simulink model "mariner_simtr"  (R2018b)
settings: Solver=FixedStepAuto  StartTime=0.0  StopTime=600  FixedStep=0.1  RelTol=1e-3
libraries: neural x211, simulink x2
(part 10 of 10)

== system mariner_simtr/NN transform (normalizing)/Layer 4/Delays 1 ==
  "p{4}" : Inport  PortDimensions=24
      mask Display: e = 0.06;c1 = [120 230 180]/255;c2 = ([120 230 180]+0)/(256+128);c3 = ([120 230 180]+128)/(256+128);patch([0 1 1 0],[0 0 1 1],c1);patch([0 1 1 1-e 1-e 0+e],[0 0 1 1-e 0+e 0+e],c2);patch([0 0 1 1-e 0+e 0+e],[0 1 1 1-e 1-e 0+e],c3);plot([0 1 1 0 0],[0 0 1 1 0]);
  mux : Mux  Inputs=1
      mask Display: e = 0.06;c1 = [120 150 230]/255;c2 = ([120 150 230]+0)/383;c3 = ([120 150 230]+128)/383;patch([0 1 1 0],[0 0 1 1],c1);patch([0 1 1 1-e 1-e 0+e],[0 0 1 1-e 0+e 0+e],c2);patch([0 0 1 1-e 0+e 0+e],[0 1 1 1-e 1-e 0+e],c3);plot([0 1 1 0 0],[0 0 1 1 0]);disp('Mux')
  "pd{4,3}" : Outport
      mask Display: e = 0.06;c1 = [120 230 180]/255;c2 = ([120 230 180]+0)/(256+128);c3 = ([120 230 180]+128)/(256+128);patch([0 1 1 0],[0 0 1 1],c1);patch([0 1 1 1-e 1-e 0+e],[0 0 1 1-e 0+e 0+e],c2);patch([0 0 1 1-e 0+e 0+e],[0 1 1 1-e 1-e 0+e],c3);plot([0 1 1 0 0],[0 0 1 1 0]);
  wires:
  mux/1 -> "pd{4,3}"/1
  "p{4}"/1 -> mux/1

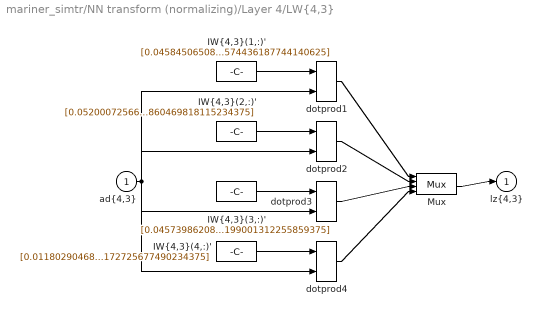
== system mariner_simtr/NN transform (normalizing)/Layer 4/LW{4,3} ==
  "ad{4,3}" : Inport  PortDimensions=24
      mask Display: e = 0.06;c1 = [120 230 180]/255;c2 = ([120 230 180]+0)/(256+128);c3 = ([120 230 180]+128)/(256+128);patch([0 1 1 0],[0 0 1 1],c1);patch([0 1 1 1-e 1-e 0+e],[0 0 1 1-e 0+e 0+e],c2);patch([0 0 1 1-e 0+e 0+e],[0 1 1 1-e 1-e 0+e],c3);plot([0 1 1 0 0],[0 0 1 1 0]);
  "IW{4,3}(1,:)'" : Constant  Value=[0.045845065089835712601740169702679850161075592041015625;0;0;0.03200214846035269455892802170637878589332103729248046875;0.002146566416768539743709087730394458048976957798004150390625;-0.00879816658090023552551972585433759377337992191314697265625;0;0;-0.00557755254364065110317394413641522987745702266693115234375;0;0;0.02027157586876295047861873399597243405878543853759765625;0;-0.01180008817101071451338700768474154756404459476470947265625;0.11876238646713321855941103422082960605621337890625;0;0.10359225441360649100364099695070763118565082550048828125;0.048299592166740783205636233788027311675250530242919921875;0;0;0;0.106186312519840730939080231109983287751674652099609375;0;-0.056572719355765667403890262221466400660574436187744140625]
      mask Display: e = 0.06;c1 = [120 150 230]/255;c2 = ([120 150 230]+0)/383;c3 = ([120 150 230]+128)/383;patch([0 1 1 0],[0 0 1 1],c1);patch([0 1 1 1-e 1-e 0+e],[0 0 1 1-e 0+e 0+e],c2);patch([0 0 1 1-e 0+e 0+e],[0 1 1 1-e 1-e 0+e],c3);plot([0 1 1 0 0],[0 0 1 1 0]);disp('weights');
  "IW{4,3}(2,:)'" : Constant  Value=[0.05200072566134460172460052262977114878594875335693359375;0;0;0.0216832850043054033151168624726778944022953510284423828125;0.006388620249107585490067062750085824518464505672454833984375;0.0030690164066453349579755016662829802953638136386871337890625;0;0;0.047402164595837119331900311181016149930655956268310546875;0;0;-0.00432370043961927651154919516329755424521863460540771484375;0;0.016146732051787272832488184803878539241850376129150390625;0.014518178667154511829462393279754905961453914642333984375;0;0.0644925875267555459569024378652102313935756683349609375;0.0163869072938503355929551474901018082164227962493896484375;0;0;0;0.049205427055631377475375387575695640407502651214599609375;0;0.0892949095175198104268332599531277082860469818115234375]
      mask Display: e = 0.06;c1 = [120 150 230]/255;c2 = ([120 150 230]+0)/383;c3 = ([120 150 230]+128)/383;patch([0 1 1 0],[0 0 1 1],c1);patch([0 1 1 1-e 1-e 0+e],[0 0 1 1-e 0+e 0+e],c2);patch([0 0 1 1-e 0+e 0+e],[0 1 1 1-e 1-e 0+e],c3);plot([0 1 1 0 0],[0 0 1 1 0]);disp('weights');
  "IW{4,3}(3,:)'" : Constant  Value=[0.045739862082544484322976785506398300640285015106201171875;0;0;0.015289627204140281147015656415533157996833324432373046875;0.006186692798785690949880944344840827398002147674560546875;0.0063214812297217766456913778938542236573994159698486328125;0;0;0.0549909753244011145767444759258069097995758056640625;0;0;-0.01041052602636438617622616220614872872829437255859375;0;0.0224029830806876974202968000327018671669065952301025390625;-0.0178193563740065286093994245675276033580303192138671875;0;0.042633639054904727549999421398752019740641117095947265625;0.00488897423933244527904928844463938730768859386444091796875;0;0;0;0.0234849334691184241652450737092294730246067047119140625;0;0.1170770490445323941397504086125991307199001312255859375]
      mask Display: e = 0.06;c1 = [120 150 230]/255;c2 = ([120 150 230]+0)/383;c3 = ([120 150 230]+128)/383;patch([0 1 1 0],[0 0 1 1],c1);patch([0 1 1 1-e 1-e 0+e],[0 0 1 1-e 0+e 0+e],c2);patch([0 0 1 1-e 0+e 0+e],[0 1 1 1-e 1-e 0+e],c3);plot([0 1 1 0 0],[0 0 1 1 0]);disp('weights');
  "IW{4,3}(4,:)'" : Constant  Value=[0.0118029046884731980693317154873511753976345062255859375;0;0;0.0033417062363545308421863833103770957677625119686126708984375;0.00147619294632471615737190351325125448056496679782867431640625;0.002331646626337603896150785232066482421942055225372314453125;0;0;0.0160008163637084289965262229316067532636225223541259765625;0;0;-0.0035403191334323793997007623346462423796765506267547607421875;0;0.007299448452192187387910227158727138885296881198883056640625;-0.00917205000330689919352256112006216426379978656768798828125;0;0.00859965631528962319574116435205723973922431468963623046875;-4.6966271232805716626980407912839154960238374769687652587890625e-05;0;0;0;0.0023517992026062285726428768839468830265104770660400390625;0;0.03575048802612511289478192111346288584172725677490234375]
      mask Display: e = 0.06;c1 = [120 150 230]/255;c2 = ([120 150 230]+0)/383;c3 = ([120 150 230]+128)/383;patch([0 1 1 0],[0 0 1 1],c1);patch([0 1 1 1-e 1-e 0+e],[0 0 1 1-e 0+e 0+e],c2);patch([0 0 1 1-e 0+e 0+e],[0 1 1 1-e 1-e 0+e],c3);plot([0 1 1 0 0],[0 0 1 1 0]);disp('weights');
  Mux : Mux
      mask Display: e = 0.06;c1 = [120 150 230]/255;c2 = ([120 150 230]+0)/383;c3 = ([120 150 230]+128)/383;patch([0 1 1 0],[0 0 1 1],c1);patch([0 1 1 1-e 1-e 0+e],[0 0 1 1-e 0+e 0+e],c2);patch([0 0 1 1-e 0+e 0+e],[0 1 1 1-e 1-e 0+e],c3);plot([0 1 1 0 0],[0 0 1 1 0]);disp('Mux');
  dotprod{1..4} (4 alike) : neural/Weight Functions/dotprod
  "lz{4,3}" : Outport
      mask Display: e = 0.06;c1 = [120 230 180]/255;c2 = ([120 230 180]+0)/(256+128);c3 = ([120 230 180]+128)/(256+128);patch([0 1 1 0],[0 0 1 1],c1);patch([0 1 1 1-e 1-e 0+e],[0 0 1 1-e 0+e 0+e],c2);patch([0 0 1 1-e 0+e 0+e],[0 1 1 1-e 1-e 0+e],c3);plot([0 1 1 0 0],[0 0 1 1 0]);
  wires:
  Mux/1 -> "lz{4,3}"/1
  dotprod4/1 -> Mux/4
  "IW{4,3}(4,:)'"/1 -> dotprod4/1
  dotprod3/1 -> Mux/3
  "IW{4,3}(3,:)'"/1 -> dotprod3/1
  dotprod2/1 -> Mux/2
  "IW{4,3}(2,:)'"/1 -> dotprod2/1
  dotprod1/1 -> Mux/1
  "ad{4,3}"/1 -> dotprod4/2, dotprod3/2, dotprod2/2, dotprod1/2
  "IW{4,3}(1,:)'"/1 -> dotprod1/1

== matlab function mariner_simtr/MATLAB Function1 ==
  data: u input; y output
function y = fcn(u)
%Define constants
max_X = 2.7814e-06; min_X = -1.0709e-05;
max_U = 7.7175; min_U = 7.6988;
max_Y = 1.5709e-04; min_Y = -3.4372e-04;
max_N = 1.1898e-04; min_N = -2.4995e-05;
%Denormalize outputs
y = zeros(1,4);
y(1) = u(1)*(max_U-min_U)+min_U;
y(2) = u(2)*(max_X-min_X)+min_X;
y(3) = u(3)*(max_Y-min_Y)+min_Y;
y(4) = u(4)*(max_N-min_N)+min_N;

== matlab function mariner_simtr/MATLAB Function ==
  data: u input; y output
function y = fcn(u)
%Write down constants to be used for normalization of states
max_u = 0.0; min_u = -0.0192;
max_v = 0.0372; min_v = -0.1668;
max_r = 0.0029; min_r = -4.9078e-04;
max_x = 4.6013e+03; min_x = 0;
max_y = 476.7522; min_y = -0.0323;
max_psi = 0.1295; min_psi = 0;
max_delta = 0.0445; min_delta = -0.0779;
%Compute the outputs
y = zeros(7,1); %Initialize output vector
y(1) = (u(1) -min_u)/(max_u - min_u);
y(2) = (u(2) -min_v)/(max_v - min_v);
y(3) = (u(3) -min_r)/(max_r - min_r);
y(4) = (u(4) -min_x)/(max_x - min_x);
y(5) = (u(5) -min_y)/(max_y - min_y);
y(6) = (u(6) -min_psi)/(max_psi - min_psi);
y(7) = (u(7) -min_delta)/(max_delta - min_delta);

== stateflow chart mariner_simtr/mariner ==
  settings: updateMethod=CONTINUOUS
  state xdot
    en:
    m11 = 0.0084;
    m32 = -2.3000e-04;
    m33 = 8.3000e-04;
    m23 = -9.0000e-05;
    m22 = 0.0155;
    detM22 = 1.2811e-05;
    L = 160.93;
    if abs(ui) >= 40*pi/180,
    delta_c = sign(-ui)*40*pi/180;
    else,
    delta_c = -ui;
    end
    du:
    %States
    u_dot = X*(U^2/L)/m11;
    v_dot = -(-m33*Y+m23*N)*(U^2/L)/detM22;
    r_dot = (-m32*Y+m22*N)*(U^2/L^2)/detM22;
    x_dot = (cos(psi)*(U0/U+u)-sin(psi)*v)*U;
    y_dot = (sin(psi)*(U0/U+u)+cos(psi)*v)*U;
    psi_dot = r*(U/L);
    delta_dot = max(min(delta_c - delta,5*pi/180),-5*pi/180);
    %Outputs
    u_out = u;
    v_out = v;
    r_out = r;
    x_out = x;
    y_out = y;
    psi_out = psi;
    delta_out = delta;
  (default) -> xdot : {u=0.0;
      | v = 0;
      | r = 0;
      | x = 0;
      | y = 0;
      | psi = 0;
      | delta = 0;}
  data: U input; u_out output; detM22 local double; v_out output; r_out output; x_out output; y_out output; psi_out output; delta_out output; delta_c local; u local; psi local; v local; r local; x local; delta local; y local; m22 local double; m11 local double; m33 local double; m32 local double; m23 local double; X input; Y input; L local double; N input; ui input; U0 constant double
  data u settings: updateMethod=SF_CONTINUOUS_TIME_DATA
  data psi settings: updateMethod=SF_CONTINUOUS_TIME_DATA
  data v settings: updateMethod=SF_CONTINUOUS_TIME_DATA
  data r settings: updateMethod=SF_CONTINUOUS_TIME_DATA
  data x settings: updateMethod=SF_CONTINUOUS_TIME_DATA
  data delta settings: updateMethod=SF_CONTINUOUS_TIME_DATA
  data y settings: updateMethod=SF_CONTINUOUS_TIME_DATA
